simulink model "R7014E_QuadTankSim"  (R2018b)
settings: Solver=ode4  StartTime=0.0  StopTime=200  FixedStep=0.01  RelTol=1e-3  EnableMultiTasking=on
undefined symbols (not defined in the file or in its folder): den, den2, num, num2, sigbuilder_block
libraries: simulink x2
Description:
  | Double tank process simulation model
  | V1.0
  | 
  | Author: Wolfgang Birk, LTU
settings Model: MinMaxOverflowLogging=ForceOff  Creator=wolfgang  LastModifiedBy=OscarBackman
settings DataIOCC: LimitDataPoints=on  SaveFormat=Array  SignalLoggingSaveFormat=ModelDataLogs
settings OptimizationCC: ExpressionDepthLimit=2147483647  LifeSpan=inf
settings DebuggingCC: UnderspecifiedInitializationDetection=Classic  MergeDetectMultiDrivingBlocksExec=none  SolverPrmCheckMsg=warning  FcnCallInpInsideContextMsg=warning  StateNameClashWarn=warning  LibraryContextMissingDiagnostic=none  SFUnexpectedBacktrackingDiag=warning  SFNoUnconditionalDefaultTransitionDiag=warning  SFExecutionAtInitializationDiag=none
settings HardwareCC: ProdBitPerPointer=32  ProdBitPerSizeT=32  ProdBitPerPtrDiffT=32  ProdLargestAtomicFloat=None  ProdIntDivRoundTo=Undefined  ProdEndianess=Unspecified  ProdWordSize=32  ProdHWDeviceType=32-bit Generic
settings ModelReferenceCC: PropagateSignalLabelsOutOfModel=off
settings SFSimCC: SimUseLocalCustomCode=off
settings RTWCC: RTWUseLocalCustomCode=off
settings CodeAppCC: StateflowObjectComments=on
settings GRTTargetCC: TargetLangStandard=C89/C90 (ANSI)  GeneratePreprocessorConditionals=Disable all
settings ConfigComp: CovMetricSettings=dw  CovHtmlReporting=on  CovSaveCumulativeToWorkspaceVar=on  CovSaveSingleToWorkspaceVar=on  CovExternalEMLEnable=off

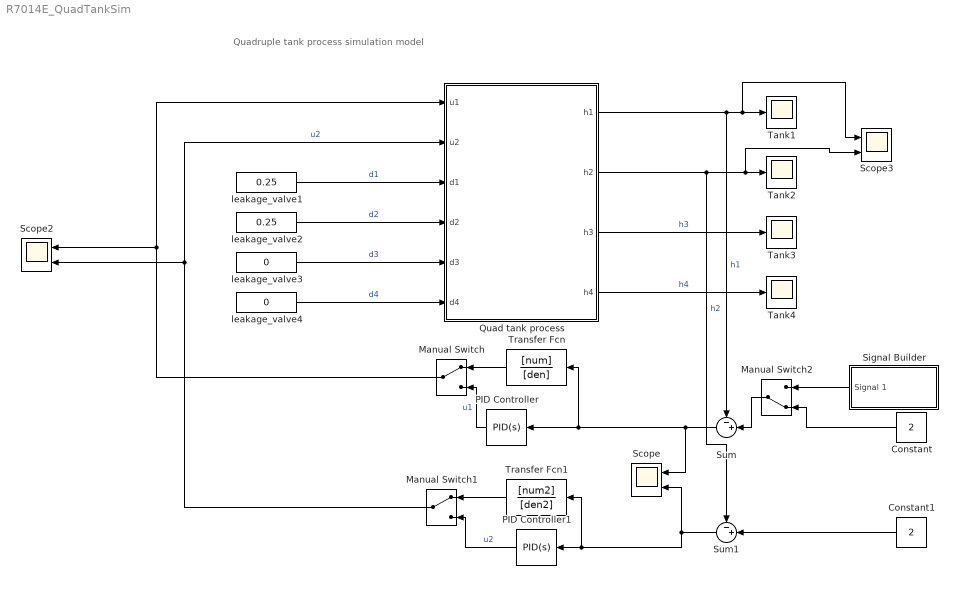
== system R7014E_QuadTankSim ==
  note: Quadruple tank process simulation model
  Constant : Constant  Value=2
  Constant1 : Constant  Value=2
  Manual Switch : ManualSwitch
  Manual Switch1 : ManualSwitch
  Manual Switch2 : ManualSwitch  CurrentSetting=0
  PID Controller : simulink/Continuous/PID Controller  Controller=PID  Form=Parallel  TimeDomain=Continuous-time  SampleTime=-1  IntegratorMethod=Forward Euler  FilterMethod=Forward Euler  ControllerParametersSource=internal  P=5  I=0.1  D=0  UseFilter=on  N=100  TunerSelectOption=Transfer Function Based (PID Tuner App)  InitialConditionSource=internal  InitialConditionForIntegrator=0  InitialConditionForFilter=0  DifferentiatorICPrevScaledInput=0  ExternalReset=none  TrackingMode=off  Kt=1  LimitOutput=off  UpperSaturationLimit=inf  LowerSaturationLimit=-inf  LinearizeAsGain=on  AntiWindupMode=none  Kb=1  POutMin=[]  POutMax=[]  IOutMin=[]  IOutMax=[]  DOutMin=[]  DOutMax=[]  NOutMin=[]  NOutMax=[]  SumOutMin=[]  SumOutMax=[]  SaturationOutMin=[]  SaturationOutMax=[]  PParamMin=[]  PParamMax=[]  IParamMin=[]  IParamMax=[]  DParamMin=[]  DParamMax=[]  NParamMin=[]  NParamMax=[]  KbParamMin=[]  KbParamMax=[]  KtParamMin=[]  KtParamMax=[]  KbOutMin=[]  KbOutMax=[]  KtOutMin=[]  KtOutMax=[]  IntegratorOutMin=[]  IntegratorOutMax=[]  FilterOutMin=[]  FilterOutMax=[]  SumI1OutMin=[]  SumI1OutMax=[]  SumI2OutMin=[]  SumI2OutMax=[]  SumI3OutMin=[]  SumI3OutMax=[]  SumI4OutMin=[]  SumI4OutMax=[]  SumDOutMin=[]  SumDOutMax=[]  DifferentiatorOutMin=[]  DifferentiatorOutMax=[]  FilterDiffOutCoefMin=[]  FilterDiffOutCoefMax=[]  ReciprocalOutMin=[]  ReciprocalOutMax=[]  SumDenOutMin=[]  SumDenOutMax=[]  SumNumOutMin=[]  SumNumOutMax=[]  DivideOutMin=[]  DivideOutMax=[]  IntegratorContinuousStateAttributes=''  IntegratorStateMustResolveToSignalObject=off  IntegratorRTWStateStorageClass=Auto  FilterContinuousStateAttributes=''  FilterStateMustResolveToSignalObject=off  FilterRTWStateStorageClass=Auto  ParallelPVariant=InternalParameters  IdealPVariant=Disabled  IVariant=InternalParameters  DVariant=InternalParameters  IntegratorVariant=Continuous  SatVariant=Disabled  AWVariant=Passthrough  PCopyVariant=Disabled  TRVariant=Disabled  FdbkBlocksVariant=Forward  IdealPFdbkVariant=Disabled  SatFdbkVariant=Disabled  DerivativeFilterVariant=ContFilter  NVariant=InternalParameters  NCopyVariant=Disabled  FilterICVariant=InternalICsFilter  IntegratorICVariant=InternalICs  ExternalResetVariant=Disabled  TRSumVariant=Passthrough  SumFdbkVariant=Disabled  SumVariant=Sum_PID
  PID Controller1 : simulink/Continuous/PID Controller  Controller=PID  Form=Parallel  TimeDomain=Continuous-time  SampleTime=-1  IntegratorMethod=Forward Euler  FilterMethod=Forward Euler  ControllerParametersSource=internal  P=2  I=0.1  D=0  UseFilter=on  N=100  TunerSelectOption=Transfer Function Based (PID Tuner App)  InitialConditionSource=internal  InitialConditionForIntegrator=0  InitialConditionForFilter=0  DifferentiatorICPrevScaledInput=0  ExternalReset=none  TrackingMode=off  Kt=1  LimitOutput=off  UpperSaturationLimit=inf  LowerSaturationLimit=-inf  LinearizeAsGain=on  AntiWindupMode=none  Kb=1  POutMin=[]  POutMax=[]  IOutMin=[]  IOutMax=[]  DOutMin=[]  DOutMax=[]  NOutMin=[]  NOutMax=[]  SumOutMin=[]  SumOutMax=[]  SaturationOutMin=[]  SaturationOutMax=[]  PParamMin=[]  PParamMax=[]  IParamMin=[]  IParamMax=[]  DParamMin=[]  DParamMax=[]  NParamMin=[]  NParamMax=[]  KbParamMin=[]  KbParamMax=[]  KtParamMin=[]  KtParamMax=[]  KbOutMin=[]  KbOutMax=[]  KtOutMin=[]  KtOutMax=[]  IntegratorOutMin=[]  IntegratorOutMax=[]  FilterOutMin=[]  FilterOutMax=[]  SumI1OutMin=[]  SumI1OutMax=[]  SumI2OutMin=[]  SumI2OutMax=[]  SumI3OutMin=[]  SumI3OutMax=[]  SumI4OutMin=[]  SumI4OutMax=[]  SumDOutMin=[]  SumDOutMax=[]  DifferentiatorOutMin=[]  DifferentiatorOutMax=[]  FilterDiffOutCoefMin=[]  FilterDiffOutCoefMax=[]  ReciprocalOutMin=[]  ReciprocalOutMax=[]  SumDenOutMin=[]  SumDenOutMax=[]  SumNumOutMin=[]  SumNumOutMax=[]  DivideOutMin=[]  DivideOutMax=[]  IntegratorContinuousStateAttributes=''  IntegratorStateMustResolveToSignalObject=off  IntegratorRTWStateStorageClass=Auto  FilterContinuousStateAttributes=''  FilterStateMustResolveToSignalObject=off  FilterRTWStateStorageClass=Auto  ParallelPVariant=InternalParameters  IdealPVariant=Disabled  IVariant=InternalParameters  DVariant=InternalParameters  IntegratorVariant=Continuous  SatVariant=Disabled  AWVariant=Passthrough  PCopyVariant=Disabled  TRVariant=Disabled  FdbkBlocksVariant=Forward  IdealPFdbkVariant=Disabled  SatFdbkVariant=Disabled  DerivativeFilterVariant=ContFilter  NVariant=InternalParameters  NCopyVariant=Disabled  FilterICVariant=InternalICsFilter  IntegratorICVariant=InternalICs  ExternalResetVariant=Disabled  TRSumVariant=Passthrough  SumFdbkVariant=Disabled  SumVariant=Sum_PID
  Quad tank process : Subsystem  mask{hmax=20, A1=28, ao1=0.071, h10=0, A2=32, ao2=0.057, h20=0, A3=28, ao3=0.071, h30=0, A4=32, ao4=0.057, h40=0, k1=3.33, k2=3.35, gamma1=0.7, gamma2=0.6}
      mask prompts: hmax "Tank height (cm)"; A1 "Tank area (cm^2)"; ao1 "Opening area (cm^2)"; h10 "Initial level (cm)"; A2 "Tank area (cm^2)"; ao2 "Opening area (cm^2)"; h20 "Initial level (cm)"; A3 "Tank area (cm^2)"; ao3 "Opening area (cm^2)"; h30 "Initial level (cm)"; A4 "Tank area (cm^2)"; ao4 "Opening area (cm^2)"; h40 "Initial level (cm)"; k1 "Pump1 gain (cm^3/V/s)"; k2 "Pump2 gain (cm^3/V/s)"; gamma1 "Split valve gamma 1"; gamma2 "Split valve gamma 2"
      mask help: Double tank process parameters
      mask DialogControl Container3 Prompt: General parameters
      mask DialogControl ParameterGroupVar Prompt: Tank 1
      mask DialogControl ParameterGroupVar_copy_copy_copy Prompt: Tank 2
      mask DialogControl ParameterGroupVar_copy_copy Prompt: Tank 3
      mask DialogControl ParameterGroupVar_copy Prompt: Tank 4
      mask DialogControl Container4 Prompt: Pump parameters
  Scope : Scope  NumInputPorts=2
  Scope2 : Scope  NumInputPorts=2
  Scope3 : Scope  NumInputPorts=2
  Signal Builder : Subsystem  Tag=STV Subsys  LoadFcn=sigbuilder_block('load');  StartFcn=sigbuilder_block('start');  StopFcn=sigbuilder_block('stop');  ClipboardFcn=sigbuilder_block('clipboard');  mask(Sigbuilder block){tuvar=[0:10]}
      mask help: Simulink:masks:SigbuilderBlock_MD
      mask init:
      | if ~strcmp(get_param(bdroot(gcbh),'SimulationStatus'),'stopped') tuvar = sigbuilder_block('maskInit'); end
      settings: CopyFcn=sigbuilder_block('copy');  DeleteFcn=sigbuilder_block('delete');  ModelCloseFcn=sigbuilder_block('modelClose');  PreSaveFcn=sigbuilder_block('preSave');  PauseFcn=sigbuilder_block('pause');  ContinueFcn=sigbuilder_block('continue');  NameChangeFcn=sigbuilder_block('namechange');  OpenFcn=sigbuilder_block('open',[431.4 178.8 550.8 400.2 ]);  CloseFcn=sigbuilder_block('close');
      mask Display: plot(0, 0, 100, 100,[2, 2, 32, 32, 2], [68, 8, 8, 68, 68],[32, 2], [38, 38], [32, 19, 2],[53, 60, 44], [32, 17, 17, 2],[16, 16, 31, 31]);txt = getActiveGroup(gcbh);text(2, 100, txt,'verticalAlignment', 'top');
  Sum : Sum  Inputs=-+|
  Sum1 : Sum  Inputs=-+|
  Tank{1..4} (4 alike) : Scope
  Transfer Fcn : TransferFcn  Numerator=[num]  Denominator=[den]
  Transfer Fcn1 : TransferFcn  Numerator=[num2]  Denominator=[den2]
  leakage_valve1 : Constant  Value=0.25
  leakage_valve2 : Constant  Value=0.25
  leakage_valve3 : Constant  Value=0
  leakage_valve4 : Constant  Value=0
  wires:
  Quad tank process/3(h3) -> Tank3/1  "h3"
  Quad tank process/1(h1) -> Sum/1, Scope3/1, Tank1/1  "h1"
  leakage_valve1/1 -> Quad tank process/3(d1)  "d1"
  leakage_valve2/1 -> Quad tank process/4(d2)  "d2"
  leakage_valve3/1 -> Quad tank process/5(d3)  "d3"
  leakage_valve4/1 -> Quad tank process/6(d4)  "d4"
  PID Controller1/1 -> Manual Switch1/2  "u2"
  Quad tank process/2(h2) -> Scope3/2, Tank2/1, Sum1/1  "h2"
  Quad tank process/4(h4) -> Tank4/1  "h4"
  Sum/1 -> Scope/1, Transfer Fcn/1, PID Controller/1
  Constant/1 -> Manual Switch2/2
  Constant1/1 -> Sum1/2
  Sum1/1 -> Scope/2, Transfer Fcn1/1, PID Controller1/1
  PID Controller/1 -> Manual Switch/2  "u1"
  Transfer Fcn/1 -> Manual Switch/1
  Manual Switch/1 -> Quad tank process/1(u1), Scope2/1
  Transfer Fcn1/1 -> Manual Switch1/1
  Manual Switch1/1 -> Scope2/2, Quad tank process/2(u2)  "u2"
  Signal Builder/1(Signal 1) -> Manual Switch2/1
  Manual Switch2/1 -> Sum/2

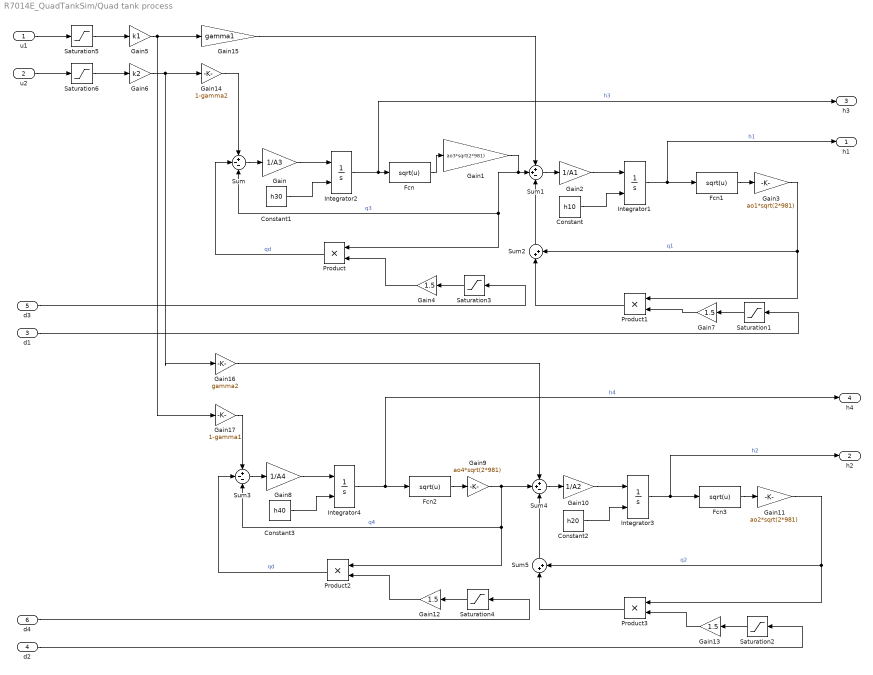
== system R7014E_QuadTankSim/Quad tank process ==
  u1 : Inport
  u2 : Inport  Port=2
  d1 : Inport  Port=3
  d2 : Inport  Port=4
  d3 : Inport  Port=5
  d4 : Inport  Port=6
  Constant : Constant  Value=h10
  Constant1 : Constant  Value=h30
  Constant2 : Constant  Value=h20
  Constant3 : Constant  Value=h40
  Fcn{,1..3} (4 alike) : Fcn  Expr=sqrt(u)
  Gain : Gain  Gain=1/A3
  Gain1 : Gain  Gain=ao3*sqrt(2*981)
  Gain10 : Gain  Gain=1/A2
  Gain11 : Gain  Gain=ao2*sqrt(2*981)
  Gain{4,7,12..13} (4 alike) : Gain  Gain=1.5
  Gain14 : Gain  Gain=1-gamma2
  Gain15 : Gain  Gain=gamma1
  Gain16 : Gain  Gain=gamma2
  Gain17 : Gain  Gain=1-gamma1
  Gain2 : Gain  Gain=1/A1
  Gain3 : Gain  Gain=ao1*sqrt(2*981)
  Gain5 : Gain  Gain=k1
  Gain6 : Gain  Gain=k2
  Gain8 : Gain  Gain=1/A4
  Gain9 : Gain  Gain=ao4*sqrt(2*981)
  Integrator{1..4} (4 alike) : Integrator  InitialConditionSource=external  LimitOutput=on  UpperSaturationLimit=hmax  LowerSaturationLimit=0
  Product{,1..3} (4 alike) : Product  RndMeth=Zero
  Saturation{1..4} (4 alike) : Saturate  UpperLimit=1  LowerLimit=0
  Saturation5 : Saturate  UpperLimit=10  LowerLimit=0
  Saturation6 : Saturate  UpperLimit=10  LowerLimit=0
  Sum : Sum  Inputs=+--
  Sum1 : Sum  Inputs=++-
  Sum2 : Sum  Inputs=|++
  Sum3 : Sum  Inputs=+--
  Sum4 : Sum  Inputs=++-
  Sum5 : Sum  Inputs=|++
  h1 : Outport
  h2 : Outport  Port=2
  h3 : Outport  Port=3
  h4 : Outport  Port=4
  wires:
  Sum/1 -> Gain/1
  Gain/1 -> Integrator2/1
  Fcn/1 -> Gain1/1
  Gain1/1 -> Product/1, Sum/3, Sum1/2  "q3"
  Sum1/1 -> Gain2/1
  Gain2/1 -> Integrator1/1
  Fcn1/1 -> Gain3/1
  Integrator2/1 -> h3/1, Fcn/1  "h3"
  Product/1 -> Sum/2  "qd"
  d3/1 -> Saturation3/1
  Integrator1/1 -> h1/1, Fcn1/1  "h1"
  Saturation3/1 -> Gain4/1
  Gain4/1 -> Product/2
  u1/1 -> Saturation5/1
  Constant/1 -> Integrator1/2
  Constant1/1 -> Integrator2/2
  u2/1 -> Saturation6/1
  Gain5/1 -> Gain17/1, Gain15/1
  Sum2/1 -> Sum1/3
  Gain3/1 -> Product1/1, Sum2/2  "q1"
  Gain7/1 -> Product1/2
  Saturation1/1 -> Gain7/1
  d1/1 -> Saturation1/1
  Product1/1 -> Sum2/1
  Product3/1 -> Sum5/1
  d2/1 -> Saturation2/1
  Saturation2/1 -> Gain13/1
  Gain13/1 -> Product3/2
  Gain11/1 -> Sum5/2, Product3/1  "q2"
  Sum5/1 -> Sum4/3
  Constant3/1 -> Integrator4/2
  Constant2/1 -> Integrator3/2
  Gain12/1 -> Product2/2
  Saturation4/1 -> Gain12/1
  Integrator3/1 -> Fcn3/1, h2/1  "h2"
  d4/1 -> Saturation4/1
  Product2/1 -> Sum3/2  "qd"
  Integrator4/1 -> h4/1, Fcn2/1  "h4"
  Fcn3/1 -> Gain11/1
  Gain10/1 -> Integrator3/1
  Sum4/1 -> Gain10/1
  Gain9/1 -> Sum4/2, Sum3/3, Product2/1  "q4"
  Fcn2/1 -> Gain9/1
  Gain8/1 -> Integrator4/1
  Sum3/1 -> Gain8/1
  Gain14/1 -> Sum/1
  Gain15/1 -> Sum1/1
  Gain6/1 -> Gain16/1, Gain14/1
  Gain16/1 -> Sum4/1
  Gain17/1 -> Sum3/1
  Saturation5/1 -> Gain5/1
  Saturation6/1 -> Gain6/1

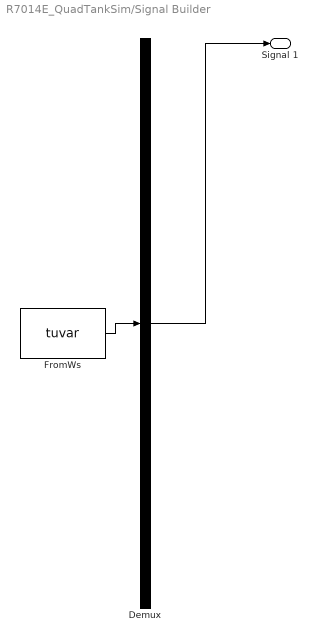
== system R7014E_QuadTankSim/Signal Builder ==
  Demux : Demux  Tag=STV Demux  Outputs=1
  FromWs : FromWorkspace  Tag=STV FromWs  VariableName=tuvar  SampleTime=0
      SigBuilderData=|
      | common.afterFinalStr = 'Extrapolate'
      | common.sampleTime = 0
      | dataSet.timeRange = [0 200]
      | dataSet.name = 'Group 1'
      | sbobj.Groups.Name = 'Group 1'
      | sbobj.Groups.Signals.Name = 'Signal 1'
      | sbobj.Groups.Signals.XData = [0 100 100 200]
      | sbobj.Groups.Signals.YData = [6 6 3 3]
      | sbobj.Groups.TimeRange = [0 200]
  Signal 1 : Outport  Tag=STV Outport
  wires:
  Demux/1 -> Signal 1/1
  FromWs/1 -> Demux/1
